simulink model "csv_planning_test"  (R2023a)
settings: configuration reference "config" (kept outside this file)
settings Model: DataDictionary=model_config.sldd  Creator=huangcheng  LastModifiedBy=Administrator
settings ConfigSetRef: SourceName=config

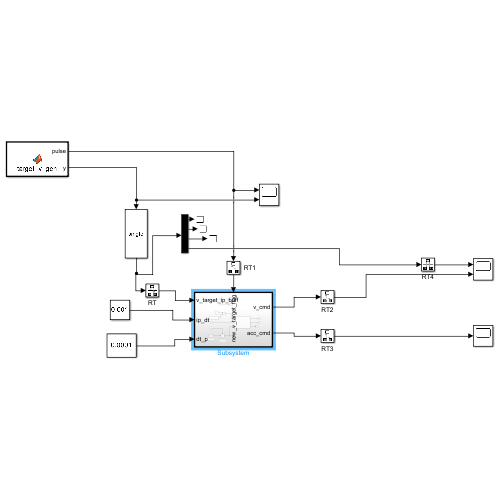
[thumbnail: Simulink's stored preview of the top-level diagram]
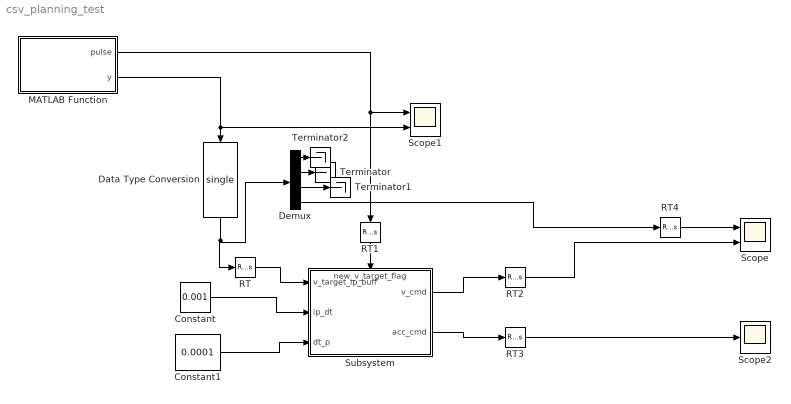
== system csv_planning_test ==
  Constant : Constant  Value=0.001  OutDataTypeStr=single
  Constant1 : Constant  Value=0.0001  OutDataTypeStr=single
  Data Type Conversion : DataTypeConversion  OutDataTypeStr=single  SaturateOnIntegerOverflow=off  RndMeth=Floor
  Demux : Demux
  MATLAB Function : MATLAB Function  TreatAsAtomicUnit=on  SystemSampleTime=1e-5
  RT{,1..4} (5 alike) : RateTransition  OutPortSampleTime=10e-5
  Scope : Scope  NumInputPorts=2
  Scope1 : Scope  NumInputPorts=2
  Scope2 : Scope
  Subsystem : Subsystem  TreatAsAtomicUnit=on  SystemSampleTime=10e-5
      settings: PortSchema="{\"entries\":[{\"content\":{\"sides\":[{\"content\":{\"connectorIds\":[\"In1\",\"In2\",\"In3\"]},\"type\":\"ConnectorPlacement.EquallySpacedRectSide\",\"uuid\":\"26201c8b-58dd-4c01-907e-9d43ba6ac588\"},{\"content\":{\"connectorIds\":[\"Out1\",\"Out2\"],\"side\":\"RIGHT\"},\"type\":\"ConnectorPlacement.EquallySpacedRectSide\",\"uuid\":\"0ccc0be0-9c4b-4afc-9c17-95ace43f2b8b\"},{\"content\":{\"connectorIds\":[\"In4\"],\"side\":\"TOP\"},\"type\":\"ConnectorPlacement.EquallySpacedRectSide\",\"uuid\":\"3f7dbbe0-0858-44b6-b8a0-1b1ed3d75812\"}]},\"type\":\"ConnectorPlacement.EquallySpacedConnector\",\"uuid\":\"a765d57e-85c3-432c-a64f-299139d869d8\"}],\"packageUris\":[\"http://schema.mathworks.com/mf0/Connector/R2020b\"],\"version\":\"1.0\"}"
  Terminator : Terminator
  Terminator1 : Terminator
  Terminator2 : Terminator
  wires:
  Constant/1 -> Subsystem/2(ip_dt)
  Constant1/1 -> Subsystem/3(dt_p)
  MATLAB Function/2(y) -> Scope1/2, Data Type Conversion/1
  MATLAB Function/1(pulse) -> RT1/1, Scope1/1
  RT2/1 -> Scope/2
  Subsystem/2(acc_cmd) -> RT3/1
  Data Type Conversion/1 -> RT/1, Demux/1
  RT/1 -> Subsystem/1(v_target_ip_buff)
  RT1/1 -> Subsystem/4(new_v_target_flag)
  Demux/2 -> Terminator/1
  Demux/3 -> Terminator1/1
  Demux/4 -> RT4/1
  Subsystem/1(v_cmd) -> RT2/1
  RT3/1 -> Scope2/1
  RT4/1 -> Scope/1
  Demux/1 -> Terminator2/1

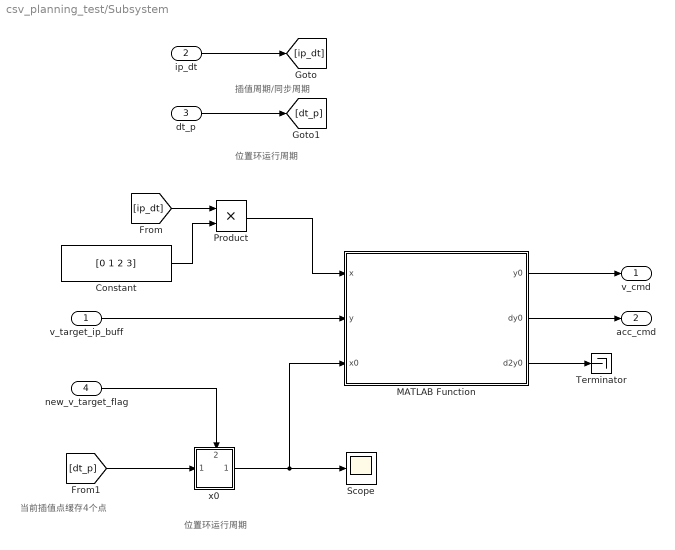
== system csv_planning_test/Subsystem ==
  note: 插值周期/同步周期
  note: 当前插值点缓存4个点
  note: 位置环运行周期
  note: 位置环运行周期
  v_target_ip_buff : Inport  OutDataTypeStr=single  PortDimensions=4
  ip_dt : Inport  Port=2
  dt_p : Inport  Port=3
  new_v_target_flag : Inport  Port=4
  Constant : Constant  Value=[0 1 2 3]  OutDataTypeStr=single
  MATLAB Function : MATLAB Function  SystemSampleTime=10e-5
  Product : Product
  Scope : Scope
  Terminator : Terminator
  x0 : Subsystem
      settings: PortSchema="{\"entries\":[{\"content\":{\"sides\":[{\"content\":{\"connectorIds\":[\"In1\"]},\"type\":\"ConnectorPlacement.EquallySpacedRectSide\",\"uuid\":\"70c20c04-e2c1-4bd3-8b77-8c863c6d80e9\"},{\"content\":{\"connectorIds\":[\"Out1\"],\"side\":\"RIGHT\"},\"type\":\"ConnectorPlacement.EquallySpacedRectSide\",\"uuid\":\"b835eda6-ef4c-4d76-aec8-67fa45d28ff2\"},{\"content\":{\"connectorIds\":[\"In2\"],\"side\":\"TOP\"},\"type\":\"ConnectorPlacement.EquallySpacedRectSide\",\"uuid\":\"c88a132b-0aa4-4cac-a486-e2b7a96ab1dd\"}]},\"type\":\"ConnectorPlacement.EquallySpacedConnector\",\"uuid\":\"c566a6b8-a329-43f5-b8b3-70b61d6d004d\"}],\"packageUris\":[\"http://schema.mathworks.com/mf0/Connector/R2020b\"],\"version\":\"1.0\"}"
  v_cmd : Outport
  acc_cmd : Outport  Port=2
  wires:
  MATLAB Function/3(d2y0) -> Terminator/1
  MATLAB Function/2(dy0) -> acc_cmd/1
  Product/1 -> MATLAB Function/1(x)
  ip_dt/1 -> [ip_dt]
  Constant/1 -> Product/2
  [ip_dt] -> Product/1
  x0/1(Out1) -> MATLAB Function/3(x0), Scope/1
  [dt_p] -> x0/1(In1)
  dt_p/1 -> [dt_p]
  MATLAB Function/1(y0) -> v_cmd/1
  v_target_ip_buff/1 -> MATLAB Function/2(y)
  new_v_target_flag/1 -> x0/2(new_v_target)

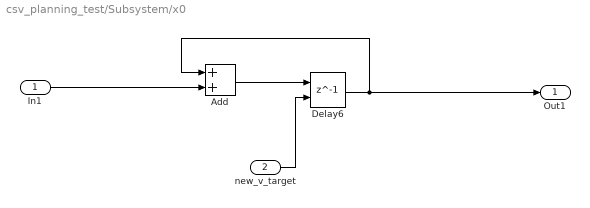
== system csv_planning_test/Subsystem/x0 ==
  In1 : Inport
  new_v_target : Inport  Port=2
  Add : Sum
  Delay6 : Delay  DelayLength=1  ExternalReset=Rising  StateName=x0_now
      settings: InputPortMap=u0,r5
  Out1 : Outport
  wires:
  In1/1 -> Add/2
  Delay6/1 -> Add/1, Out1/1
  Add/1 -> Delay6/1
  new_v_target/1 -> Delay6/2

== matlab function csv_planning_test/Subsystem/MATLAB Function ==
  data: x input; y input; y0 output; x0 input; dy0 output; d2y0 output
function [y0, dy0, d2y0]  = InterpolateSignal(x,y,x0)
 
 % 可选插值方法pchip、 makima 、spline一阶导数和二阶导数
    % 输入:
    %   pp - 返回的分段多项式结构
    %   x0 - 要计算的点（可以是向量）
    % 输出:
    %   y0  - 函数值
    %   dy0 - 一阶导数
    %   d2y0 - 二阶导数

    % 提取分段插值起点, 插值计算都减去起点
    y_init = y(1);
    yy = y - y_init;

    pp = makima(x, yy);


    % 1. 计算函数值
    y0 = ppval(pp, x0) + y_init;
    
     % 方法二：手动从系数计算
    breaks = pp.breaks;
    coefs = pp.coefs;

    %x0必须始终在插值第一段
 
    c = coefs(1, :);  % 系数为 [a, b, c, d]，对应 (x-break)^3, (x-break)^2, (x-break)^1, 常数项
    t = x0 - breaks(1);
    % 一阶导数
    dy0 = 3*c(1)*t^2 + 2*c(2)*t + c(3);
    % 二阶导数
    d2y0 = 6*c(1)*t + 2*c(2);

end

== matlab function csv_planning_test/MATLAB Function ==
  data: pulse output; y output
function [pulse, y]= target_v_gen( )

dt = 1e-5;
w = 10;
amp = 1000;
sin_t = 2*pi/w;

time_ip = 100;  %每100个周期dt 发送一次目标速度  即 1ms 发送一次

persistent y_buff t time_count 

if isempty(y_buff)
    y_buff = zeros(1, 4);
    t = 0;
    time_count = 0;

end

y0 = amp*sin(w*t);  %一直更新
t = t + dt;

if t >= sin_t
    t = t - sin_t;
end


if time_count >= time_ip  %发送一次目标位置  1ms周期
    time_count = 0;

    y_buff(1) = y_buff(2);
    y_buff(2) = y_buff(3);
    y_buff(3) = y_buff(4);
    y_buff(4) = y0;
    pulse = 1;
else 
    pulse = 1;
    if time_count >= time_ip*0.5
        pulse = 0;
    end
end
time_count = time_count + 1;

y = y_buff;
